simulink model "pde"  (Simulink 6.5)
settings: Solver=ode45  StartTime=0.0  StopTime=10.0  RelTol=1e-3
undefined symbols (not defined in the file): dfilt
libraries: dsparch4 x158, cdsEpicsOut x39, cdsMatrix x11, cdsSwitch x5, cdsWD x5, cdsWfsPhase x4, cdsEpicsIn x4, dac x2, cdsRemoteIntlk x1, cdsParameters x1
(part 2 of 3)

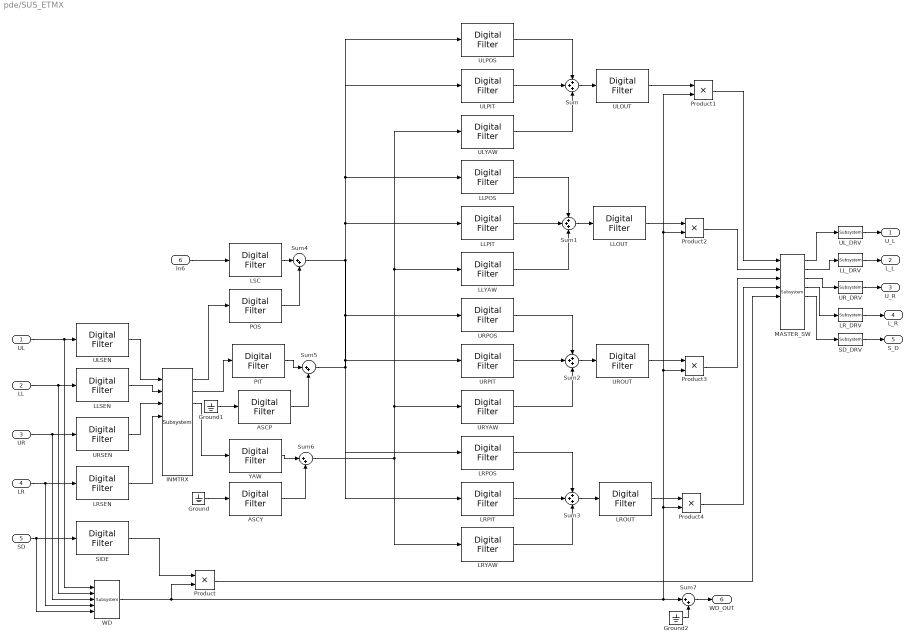
== system pde/SUS_ETMX ==
  UL : Inport
  LL : Inport  Port=2
  UR : Inport  Port=3
  LR : Inport  Port=4
  SD : Inport  Port=5
  In6 : Inport  Port=6
  ASCP : dsparch4/Digital Filter  DialogController=dspdialog.DigitalFilter  DialogControllerArgs=DataTag50  TypePopup=IIR (poles & zeros)  IIRFiltStruct=Direct form II transposed  AllPoleFiltStruct=Direct form  FIRFiltStruct=Direct form  CoeffSource=Specify via dialog  NumCoeffs=[1 2]  DenCoeffs=[1 0.1]  BiQuadCoeffs=[1 0.3 0.4 1 0.1 0.2]  LatticeCoeffs=[0.2 0.4]  denIgnore=on  FiltPerSampPopup=One filter per frame  IC=0  ICnum=0  ICden=0  roundingMode=Floor  overflowMode=off  ScaleValues=1  scaleValueFracLength=14  stageInFracLength=15  stageOutFracLength=15  FilterSource=Specify via dialog  dfiltObjectName=dfilt.dffir([1 2 1])
  ASCY : dsparch4/Digital Filter  DialogController=dspdialog.DigitalFilter  DialogControllerArgs=DataTag51  TypePopup=IIR (poles & zeros)  IIRFiltStruct=Direct form II transposed  AllPoleFiltStruct=Direct form  FIRFiltStruct=Direct form  CoeffSource=Specify via dialog  NumCoeffs=[1 2]  DenCoeffs=[1 0.1]  BiQuadCoeffs=[1 0.3 0.4 1 0.1 0.2]  LatticeCoeffs=[0.2 0.4]  denIgnore=on  FiltPerSampPopup=One filter per frame  IC=0  ICnum=0  ICden=0  roundingMode=Floor  overflowMode=off  ScaleValues=1  scaleValueFracLength=14  stageInFracLength=15  stageOutFracLength=15  FilterSource=Specify via dialog  dfiltObjectName=dfilt.dffir([1 2 1])
  Ground : Ground
  Ground1 : Ground
  Ground2 : Ground
  INMTRX : cdsMatrix/Subsystem  Tag=Matrix  Description=|  SystemSampleTime=-1
      | Purpose:                                                                 
      | Provide a matrix multiplication function for up to 8 input and 8 outputs.
      settings: AttributesFormatString=%<Tag>
  LLOUT : dsparch4/Digital Filter  DialogController=dspdialog.DigitalFilter  DialogControllerArgs=DataTag52  TypePopup=IIR (poles & zeros)  IIRFiltStruct=Direct form II transposed  AllPoleFiltStruct=Direct form  FIRFiltStruct=Direct form  CoeffSource=Specify via dialog  NumCoeffs=[1 2]  DenCoeffs=[1 0.1]  BiQuadCoeffs=[1 0.3 0.4 1 0.1 0.2]  LatticeCoeffs=[0.2 0.4]  denIgnore=on  FiltPerSampPopup=One filter per frame  IC=0  ICnum=0  ICden=0  roundingMode=Floor  overflowMode=off  ScaleValues=1  scaleValueFracLength=14  stageInFracLength=15  stageOutFracLength=15  FilterSource=Specify via dialog  dfiltObjectName=dfilt.dffir([1 2 1])
  LLPIT : dsparch4/Digital Filter  DialogController=dspdialog.DigitalFilter  DialogControllerArgs=DataTag53  TypePopup=IIR (poles & zeros)  IIRFiltStruct=Direct form II transposed  AllPoleFiltStruct=Direct form  FIRFiltStruct=Direct form  CoeffSource=Specify via dialog  NumCoeffs=[1 2]  DenCoeffs=[1 0.1]  BiQuadCoeffs=[1 0.3 0.4 1 0.1 0.2]  LatticeCoeffs=[0.2 0.4]  denIgnore=on  FiltPerSampPopup=One filter per frame  IC=0  ICnum=0  ICden=0  roundingMode=Floor  overflowMode=off  ScaleValues=1  scaleValueFracLength=14  stageInFracLength=15  stageOutFracLength=15  FilterSource=Specify via dialog  dfiltObjectName=dfilt.dffir([1 2 1])
  LLPOS : dsparch4/Digital Filter  DialogController=dspdialog.DigitalFilter  DialogControllerArgs=DataTag54  TypePopup=IIR (poles & zeros)  IIRFiltStruct=Direct form II transposed  AllPoleFiltStruct=Direct form  FIRFiltStruct=Direct form  CoeffSource=Specify via dialog  NumCoeffs=[1 2]  DenCoeffs=[1 0.1]  BiQuadCoeffs=[1 0.3 0.4 1 0.1 0.2]  LatticeCoeffs=[0.2 0.4]  denIgnore=on  FiltPerSampPopup=One filter per frame  IC=0  ICnum=0  ICden=0  roundingMode=Floor  overflowMode=off  ScaleValues=1  scaleValueFracLength=14  stageInFracLength=15  stageOutFracLength=15  FilterSource=Specify via dialog  dfiltObjectName=dfilt.dffir([1 2 1])
  LLSEN : dsparch4/Digital Filter  DialogController=dspdialog.DigitalFilter  DialogControllerArgs=DataTag55  TypePopup=IIR (poles & zeros)  IIRFiltStruct=Direct form II transposed  AllPoleFiltStruct=Direct form  FIRFiltStruct=Direct form  CoeffSource=Specify via dialog  NumCoeffs=[1 2]  DenCoeffs=[1 0.1]  BiQuadCoeffs=[1 0.3 0.4 1 0.1 0.2]  LatticeCoeffs=[0.2 0.4]  denIgnore=on  FiltPerSampPopup=One filter per frame  IC=0  ICnum=0  ICden=0  roundingMode=Floor  overflowMode=off  ScaleValues=1  scaleValueFracLength=14  stageInFracLength=15  stageOutFracLength=15  FilterSource=Specify via dialog  dfiltObjectName=dfilt.dffir([1 2 1])
  LLYAW : dsparch4/Digital Filter  DialogController=dspdialog.DigitalFilter  DialogControllerArgs=DataTag56  TypePopup=IIR (poles & zeros)  IIRFiltStruct=Direct form II transposed  AllPoleFiltStruct=Direct form  FIRFiltStruct=Direct form  CoeffSource=Specify via dialog  NumCoeffs=[1 2]  DenCoeffs=[1 0.1]  BiQuadCoeffs=[1 0.3 0.4 1 0.1 0.2]  LatticeCoeffs=[0.2 0.4]  denIgnore=on  FiltPerSampPopup=One filter per frame  IC=0  ICnum=0  ICden=0  roundingMode=Floor  overflowMode=off  ScaleValues=1  scaleValueFracLength=14  stageInFracLength=15  stageOutFracLength=15  FilterSource=Specify via dialog  dfiltObjectName=dfilt.dffir([1 2 1])
  LL_DRV : cdsEpicsOut/Subsystem  SystemSampleTime=-1
  LROUT : dsparch4/Digital Filter  DialogController=dspdialog.DigitalFilter  DialogControllerArgs=DataTag57  TypePopup=IIR (poles & zeros)  IIRFiltStruct=Direct form II transposed  AllPoleFiltStruct=Direct form  FIRFiltStruct=Direct form  CoeffSource=Specify via dialog  NumCoeffs=[1 2]  DenCoeffs=[1 0.1]  BiQuadCoeffs=[1 0.3 0.4 1 0.1 0.2]  LatticeCoeffs=[0.2 0.4]  denIgnore=on  FiltPerSampPopup=One filter per frame  IC=0  ICnum=0  ICden=0  roundingMode=Floor  overflowMode=off  ScaleValues=1  scaleValueFracLength=14  stageInFracLength=15  stageOutFracLength=15  FilterSource=Specify via dialog  dfiltObjectName=dfilt.dffir([1 2 1])
  LRPIT : dsparch4/Digital Filter  DialogController=dspdialog.DigitalFilter  DialogControllerArgs=DataTag58  TypePopup=IIR (poles & zeros)  IIRFiltStruct=Direct form II transposed  AllPoleFiltStruct=Direct form  FIRFiltStruct=Direct form  CoeffSource=Specify via dialog  NumCoeffs=[1 2]  DenCoeffs=[1 0.1]  BiQuadCoeffs=[1 0.3 0.4 1 0.1 0.2]  LatticeCoeffs=[0.2 0.4]  denIgnore=on  FiltPerSampPopup=One filter per frame  IC=0  ICnum=0  ICden=0  roundingMode=Floor  overflowMode=off  ScaleValues=1  scaleValueFracLength=14  stageInFracLength=15  stageOutFracLength=15  FilterSource=Specify via dialog  dfiltObjectName=dfilt.dffir([1 2 1])
  LRPOS : dsparch4/Digital Filter  DialogController=dspdialog.DigitalFilter  DialogControllerArgs=DataTag59  TypePopup=IIR (poles & zeros)  IIRFiltStruct=Direct form II transposed  AllPoleFiltStruct=Direct form  FIRFiltStruct=Direct form  CoeffSource=Specify via dialog  NumCoeffs=[1 2]  DenCoeffs=[1 0.1]  BiQuadCoeffs=[1 0.3 0.4 1 0.1 0.2]  LatticeCoeffs=[0.2 0.4]  denIgnore=on  FiltPerSampPopup=One filter per frame  IC=0  ICnum=0  ICden=0  roundingMode=Floor  overflowMode=off  ScaleValues=1  scaleValueFracLength=14  stageInFracLength=15  stageOutFracLength=15  FilterSource=Specify via dialog  dfiltObjectName=dfilt.dffir([1 2 1])
  LRSEN : dsparch4/Digital Filter  DialogController=dspdialog.DigitalFilter  DialogControllerArgs=DataTag60  TypePopup=IIR (poles & zeros)  IIRFiltStruct=Direct form II transposed  AllPoleFiltStruct=Direct form  FIRFiltStruct=Direct form  CoeffSource=Specify via dialog  NumCoeffs=[1 2]  DenCoeffs=[1 0.1]  BiQuadCoeffs=[1 0.3 0.4 1 0.1 0.2]  LatticeCoeffs=[0.2 0.4]  denIgnore=on  FiltPerSampPopup=One filter per frame  IC=0  ICnum=0  ICden=0  roundingMode=Floor  overflowMode=off  ScaleValues=1  scaleValueFracLength=14  stageInFracLength=15  stageOutFracLength=15  FilterSource=Specify via dialog  dfiltObjectName=dfilt.dffir([1 2 1])
  LRYAW : dsparch4/Digital Filter  DialogController=dspdialog.DigitalFilter  DialogControllerArgs=DataTag61  TypePopup=IIR (poles & zeros)  IIRFiltStruct=Direct form II transposed  AllPoleFiltStruct=Direct form  FIRFiltStruct=Direct form  CoeffSource=Specify via dialog  NumCoeffs=[1 2]  DenCoeffs=[1 0.1]  BiQuadCoeffs=[1 0.3 0.4 1 0.1 0.2]  LatticeCoeffs=[0.2 0.4]  denIgnore=on  FiltPerSampPopup=One filter per frame  IC=0  ICnum=0  ICden=0  roundingMode=Floor  overflowMode=off  ScaleValues=1  scaleValueFracLength=14  stageInFracLength=15  stageOutFracLength=15  FilterSource=Specify via dialog  dfiltObjectName=dfilt.dffir([1 2 1])
  LR_DRV : cdsEpicsOut/Subsystem  SystemSampleTime=-1
  LSC : dsparch4/Digital Filter  DialogController=dspdialog.DigitalFilter  DialogControllerArgs=DataTag62  TypePopup=IIR (poles & zeros)  IIRFiltStruct=Direct form II transposed  AllPoleFiltStruct=Direct form  FIRFiltStruct=Direct form  CoeffSource=Specify via dialog  NumCoeffs=[1 2]  DenCoeffs=[1 0.1]  BiQuadCoeffs=[1 0.3 0.4 1 0.1 0.2]  LatticeCoeffs=[0.2 0.4]  denIgnore=on  FiltPerSampPopup=One filter per frame  IC=0  ICnum=0  ICden=0  roundingMode=Floor  overflowMode=off  ScaleValues=1  scaleValueFracLength=14  stageInFracLength=15  stageOutFracLength=15  FilterSource=Specify via dialog  dfiltObjectName=dfilt.dffir([1 2 1])
  MASTER_SW : cdsSwitch/Subsystem  SystemSampleTime=-1
  PIT : dsparch4/Digital Filter  DialogController=dspdialog.DigitalFilter  DialogControllerArgs=DataTag63  TypePopup=IIR (poles & zeros)  IIRFiltStruct=Direct form II transposed  AllPoleFiltStruct=Direct form  FIRFiltStruct=Direct form  CoeffSource=Specify via dialog  NumCoeffs=[1 2]  DenCoeffs=[1 0.1]  BiQuadCoeffs=[1 0.3 0.4 1 0.1 0.2]  LatticeCoeffs=[0.2 0.4]  denIgnore=on  FiltPerSampPopup=One filter per frame  IC=0  ICnum=0  ICden=0  roundingMode=Floor  overflowMode=off  ScaleValues=1  scaleValueFracLength=14  stageInFracLength=15  stageOutFracLength=15  FilterSource=Specify via dialog  dfiltObjectName=dfilt.dffir([1 2 1])
  POS : dsparch4/Digital Filter  DialogController=dspdialog.DigitalFilter  DialogControllerArgs=DataTag64  TypePopup=IIR (poles & zeros)  IIRFiltStruct=Direct form II transposed  AllPoleFiltStruct=Direct form  FIRFiltStruct=Direct form  CoeffSource=Specify via dialog  NumCoeffs=[1 2]  DenCoeffs=[1 0.1]  BiQuadCoeffs=[1 0.3 0.4 1 0.1 0.2]  LatticeCoeffs=[0.2 0.4]  denIgnore=on  FiltPerSampPopup=One filter per frame  IC=0  ICnum=0  ICden=0  roundingMode=Floor  overflowMode=off  ScaleValues=1  scaleValueFracLength=14  stageInFracLength=15  stageOutFracLength=15  FilterSource=Specify via dialog  dfiltObjectName=dfilt.dffir([1 2 1])
  Product{,1..4} (5 alike) : Product  RndMeth=Zero
  SD_DRV : cdsEpicsOut/Subsystem  SystemSampleTime=-1
  SIDE : dsparch4/Digital Filter  DialogController=dspdialog.DigitalFilter  DialogControllerArgs=DataTag65  TypePopup=IIR (poles & zeros)  IIRFiltStruct=Direct form II transposed  AllPoleFiltStruct=Direct form  FIRFiltStruct=Direct form  CoeffSource=Specify via dialog  NumCoeffs=[1 2]  DenCoeffs=[1 0.1]  BiQuadCoeffs=[1 0.3 0.4 1 0.1 0.2]  LatticeCoeffs=[0.2 0.4]  denIgnore=on  FiltPerSampPopup=One filter per frame  IC=0  ICnum=0  ICden=0  roundingMode=Floor  overflowMode=off  ScaleValues=1  scaleValueFracLength=14  stageInFracLength=15  stageOutFracLength=15  FilterSource=Specify via dialog  dfiltObjectName=dfilt.dffir([1 2 1])
  Sum{,1..3} (4 alike) : Sum  Inputs=+++
  Sum{4..7} (4 alike) : Sum  Inputs=|++
  ULOUT : dsparch4/Digital Filter  DialogController=dspdialog.DigitalFilter  DialogControllerArgs=DataTag66  TypePopup=IIR (poles & zeros)  IIRFiltStruct=Direct form II transposed  AllPoleFiltStruct=Direct form  FIRFiltStruct=Direct form  CoeffSource=Specify via dialog  NumCoeffs=[1 2]  DenCoeffs=[1 0.1]  BiQuadCoeffs=[1 0.3 0.4 1 0.1 0.2]  LatticeCoeffs=[0.2 0.4]  denIgnore=on  FiltPerSampPopup=One filter per frame  IC=0  ICnum=0  ICden=0  roundingMode=Floor  overflowMode=off  ScaleValues=1  scaleValueFracLength=14  stageInFracLength=15  stageOutFracLength=15  FilterSource=Specify via dialog  dfiltObjectName=dfilt.dffir([1 2 1])
  ULPIT : dsparch4/Digital Filter  DialogController=dspdialog.DigitalFilter  DialogControllerArgs=DataTag67  TypePopup=IIR (poles & zeros)  IIRFiltStruct=Direct form II transposed  AllPoleFiltStruct=Direct form  FIRFiltStruct=Direct form  CoeffSource=Specify via dialog  NumCoeffs=[1 2]  DenCoeffs=[1 0.1]  BiQuadCoeffs=[1 0.3 0.4 1 0.1 0.2]  LatticeCoeffs=[0.2 0.4]  denIgnore=on  FiltPerSampPopup=One filter per frame  IC=0  ICnum=0  ICden=0  roundingMode=Floor  overflowMode=off  ScaleValues=1  scaleValueFracLength=14  stageInFracLength=15  stageOutFracLength=15  FilterSource=Specify via dialog  dfiltObjectName=dfilt.dffir([1 2 1])
  ULPOS : dsparch4/Digital Filter  DialogController=dspdialog.DigitalFilter  DialogControllerArgs=DataTag68  TypePopup=IIR (poles & zeros)  IIRFiltStruct=Direct form II transposed  AllPoleFiltStruct=Direct form  FIRFiltStruct=Direct form  CoeffSource=Specify via dialog  NumCoeffs=[1 2]  DenCoeffs=[1 0.1]  BiQuadCoeffs=[1 0.3 0.4 1 0.1 0.2]  LatticeCoeffs=[0.2 0.4]  denIgnore=on  FiltPerSampPopup=One filter per frame  IC=0  ICnum=0  ICden=0  roundingMode=Floor  overflowMode=off  ScaleValues=1  scaleValueFracLength=14  stageInFracLength=15  stageOutFracLength=15  FilterSource=Specify via dialog  dfiltObjectName=dfilt.dffir([1 2 1])
  ULSEN : dsparch4/Digital Filter  DialogController=dspdialog.DigitalFilter  DialogControllerArgs=DataTag69  TypePopup=IIR (poles & zeros)  IIRFiltStruct=Direct form II transposed  AllPoleFiltStruct=Direct form  FIRFiltStruct=Direct form  CoeffSource=Specify via dialog  NumCoeffs=[1 2]  DenCoeffs=[1 0.1]  BiQuadCoeffs=[1 0.3 0.4 1 0.1 0.2]  LatticeCoeffs=[0.2 0.4]  denIgnore=on  FiltPerSampPopup=One filter per frame  IC=0  ICnum=0  ICden=0  roundingMode=Floor  overflowMode=off  ScaleValues=1  scaleValueFracLength=14  stageInFracLength=15  stageOutFracLength=15  FilterSource=Specify via dialog  dfiltObjectName=dfilt.dffir([1 2 1])
  ULYAW : dsparch4/Digital Filter  DialogController=dspdialog.DigitalFilter  DialogControllerArgs=DataTag70  TypePopup=IIR (poles & zeros)  IIRFiltStruct=Direct form II transposed  AllPoleFiltStruct=Direct form  FIRFiltStruct=Direct form  CoeffSource=Specify via dialog  NumCoeffs=[1 2]  DenCoeffs=[1 0.1]  BiQuadCoeffs=[1 0.3 0.4 1 0.1 0.2]  LatticeCoeffs=[0.2 0.4]  denIgnore=on  FiltPerSampPopup=One filter per frame  IC=0  ICnum=0  ICden=0  roundingMode=Floor  overflowMode=off  ScaleValues=1  scaleValueFracLength=14  stageInFracLength=15  stageOutFracLength=15  FilterSource=Specify via dialog  dfiltObjectName=dfilt.dffir([1 2 1])
  UL_DRV : cdsEpicsOut/Subsystem  SystemSampleTime=-1
  UROUT : dsparch4/Digital Filter  DialogController=dspdialog.DigitalFilter  DialogControllerArgs=DataTag71  TypePopup=IIR (poles & zeros)  IIRFiltStruct=Direct form II transposed  AllPoleFiltStruct=Direct form  FIRFiltStruct=Direct form  CoeffSource=Specify via dialog  NumCoeffs=[1 2]  DenCoeffs=[1 0.1]  BiQuadCoeffs=[1 0.3 0.4 1 0.1 0.2]  LatticeCoeffs=[0.2 0.4]  denIgnore=on  FiltPerSampPopup=One filter per frame  IC=0  ICnum=0  ICden=0  roundingMode=Floor  overflowMode=off  ScaleValues=1  scaleValueFracLength=14  stageInFracLength=15  stageOutFracLength=15  FilterSource=Specify via dialog  dfiltObjectName=dfilt.dffir([1 2 1])
  URPIT : dsparch4/Digital Filter  DialogController=dspdialog.DigitalFilter  DialogControllerArgs=DataTag72  TypePopup=IIR (poles & zeros)  IIRFiltStruct=Direct form II transposed  AllPoleFiltStruct=Direct form  FIRFiltStruct=Direct form  CoeffSource=Specify via dialog  NumCoeffs=[1 2]  DenCoeffs=[1 0.1]  BiQuadCoeffs=[1 0.3 0.4 1 0.1 0.2]  LatticeCoeffs=[0.2 0.4]  denIgnore=on  FiltPerSampPopup=One filter per frame  IC=0  ICnum=0  ICden=0  roundingMode=Floor  overflowMode=off  ScaleValues=1  scaleValueFracLength=14  stageInFracLength=15  stageOutFracLength=15  FilterSource=Specify via dialog  dfiltObjectName=dfilt.dffir([1 2 1])
  URPOS : dsparch4/Digital Filter  DialogController=dspdialog.DigitalFilter  DialogControllerArgs=DataTag73  TypePopup=IIR (poles & zeros)  IIRFiltStruct=Direct form II transposed  AllPoleFiltStruct=Direct form  FIRFiltStruct=Direct form  CoeffSource=Specify via dialog  NumCoeffs=[1 2]  DenCoeffs=[1 0.1]  BiQuadCoeffs=[1 0.3 0.4 1 0.1 0.2]  LatticeCoeffs=[0.2 0.4]  denIgnore=on  FiltPerSampPopup=One filter per frame  IC=0  ICnum=0  ICden=0  roundingMode=Floor  overflowMode=off  ScaleValues=1  scaleValueFracLength=14  stageInFracLength=15  stageOutFracLength=15  FilterSource=Specify via dialog  dfiltObjectName=dfilt.dffir([1 2 1])
  URSEN : dsparch4/Digital Filter  DialogController=dspdialog.DigitalFilter  DialogControllerArgs=DataTag74  TypePopup=IIR (poles & zeros)  IIRFiltStruct=Direct form II transposed  AllPoleFiltStruct=Direct form  FIRFiltStruct=Direct form  CoeffSource=Specify via dialog  NumCoeffs=[1 2]  DenCoeffs=[1 0.1]  BiQuadCoeffs=[1 0.3 0.4 1 0.1 0.2]  LatticeCoeffs=[0.2 0.4]  denIgnore=on  FiltPerSampPopup=One filter per frame  IC=0  ICnum=0  ICden=0  roundingMode=Floor  overflowMode=off  ScaleValues=1  scaleValueFracLength=14  stageInFracLength=15  stageOutFracLength=15  FilterSource=Specify via dialog  dfiltObjectName=dfilt.dffir([1 2 1])
  URYAW : dsparch4/Digital Filter  DialogController=dspdialog.DigitalFilter  DialogControllerArgs=DataTag75  TypePopup=IIR (poles & zeros)  IIRFiltStruct=Direct form II transposed  AllPoleFiltStruct=Direct form  FIRFiltStruct=Direct form  CoeffSource=Specify via dialog  NumCoeffs=[1 2]  DenCoeffs=[1 0.1]  BiQuadCoeffs=[1 0.3 0.4 1 0.1 0.2]  LatticeCoeffs=[0.2 0.4]  denIgnore=on  FiltPerSampPopup=One filter per frame  IC=0  ICnum=0  ICden=0  roundingMode=Floor  overflowMode=off  ScaleValues=1  scaleValueFracLength=14  stageInFracLength=15  stageOutFracLength=15  FilterSource=Specify via dialog  dfiltObjectName=dfilt.dffir([1 2 1])
  UR_DRV : cdsEpicsOut/Subsystem  SystemSampleTime=-1
  WD : cdsWD/Subsystem  SystemSampleTime=-1
  YAW : dsparch4/Digital Filter  DialogController=dspdialog.DigitalFilter  DialogControllerArgs=DataTag76  TypePopup=IIR (poles & zeros)  IIRFiltStruct=Direct form II transposed  AllPoleFiltStruct=Direct form  FIRFiltStruct=Direct form  CoeffSource=Specify via dialog  NumCoeffs=[1 2]  DenCoeffs=[1 0.1]  BiQuadCoeffs=[1 0.3 0.4 1 0.1 0.2]  LatticeCoeffs=[0.2 0.4]  denIgnore=on  FiltPerSampPopup=One filter per frame  IC=0  ICnum=0  ICden=0  roundingMode=Floor  overflowMode=off  ScaleValues=1  scaleValueFracLength=14  stageInFracLength=15  stageOutFracLength=15  FilterSource=Specify via dialog  dfiltObjectName=dfilt.dffir([1 2 1])
  U_L : Outport
  L_L : Outport  Port=2
  U_R : Outport  Port=3
  L_R : Outport  Port=4
  S_D : Outport  Port=5
  WD_OUT : Outport  Port=6
  wires:
  ULSEN/1 -> INMTRX/1
  LLSEN/1 -> INMTRX/2
  URSEN/1 -> INMTRX/3
  LRSEN/1 -> INMTRX/4
  INMTRX/1 -> POS/1
  INMTRX/2 -> PIT/1
  INMTRX/3 -> YAW/1
  ULPOS/1 -> Sum/1
  ULPIT/1 -> Sum/2
  ULYAW/1 -> Sum/3
  LLPOS/1 -> Sum1/1
  LLPIT/1 -> Sum1/2
  LLYAW/1 -> Sum1/3
  URPOS/1 -> Sum2/1
  URPIT/1 -> Sum2/2
  URYAW/1 -> Sum2/3
  LRPOS/1 -> Sum3/1
  LRPIT/1 -> Sum3/2
  LRYAW/1 -> Sum3/3
  Sum/1 -> ULOUT/1
  Sum1/1 -> LLOUT/1
  Sum2/1 -> UROUT/1
  Sum3/1 -> LROUT/1
  UL/1 -> ULSEN/1, WD/1
  LL/1 -> LLSEN/1, WD/2
  UR/1 -> URSEN/1, WD/3
  LR/1 -> LRSEN/1, WD/4
  Ground1/1 -> ASCP/1
  In6/1 -> LSC/1
  Ground/1 -> ASCY/1
  LSC/1 -> Sum4/1
  POS/1 -> Sum4/2
  PIT/1 -> Sum5/1
  ASCP/1 -> Sum5/2
  YAW/1 -> Sum6/1
  ASCY/1 -> Sum6/2
  Sum4/1 -> ULPOS/1, LLPOS/1, URPOS/1, LRPOS/1
  Sum5/1 -> ULPIT/1, LLPIT/1, URPIT/1, LRPIT/1
  Sum6/1 -> ULYAW/1, LLYAW/1, URYAW/1, LRYAW/1
  SD/1 -> SIDE/1, WD/5
  WD/1 -> Product/2, Product4/2, Product3/2, Product2/2, Product1/2, Sum7/1
  SIDE/1 -> Product/1
  ULOUT/1 -> Product1/1
  LLOUT/1 -> Product2/1
  UROUT/1 -> Product3/1
  LROUT/1 -> Product4/1
  LL_DRV/1 -> L_L/1
  UL_DRV/1 -> U_L/1
  UR_DRV/1 -> U_R/1
  LR_DRV/1 -> L_R/1
  SD_DRV/1 -> S_D/1
  Product1/1 -> MASTER_SW/1
  Product2/1 -> MASTER_SW/2
  Product3/1 -> MASTER_SW/3
  Product4/1 -> MASTER_SW/4
  Product/1 -> MASTER_SW/5
  MASTER_SW/1 -> UL_DRV/1
  MASTER_SW/2 -> LL_DRV/1
  MASTER_SW/3 -> UR_DRV/1
  MASTER_SW/4 -> LR_DRV/1
  MASTER_SW/5 -> SD_DRV/1
  Sum7/1 -> WD_OUT/1
  Ground2/1 -> Sum7/2

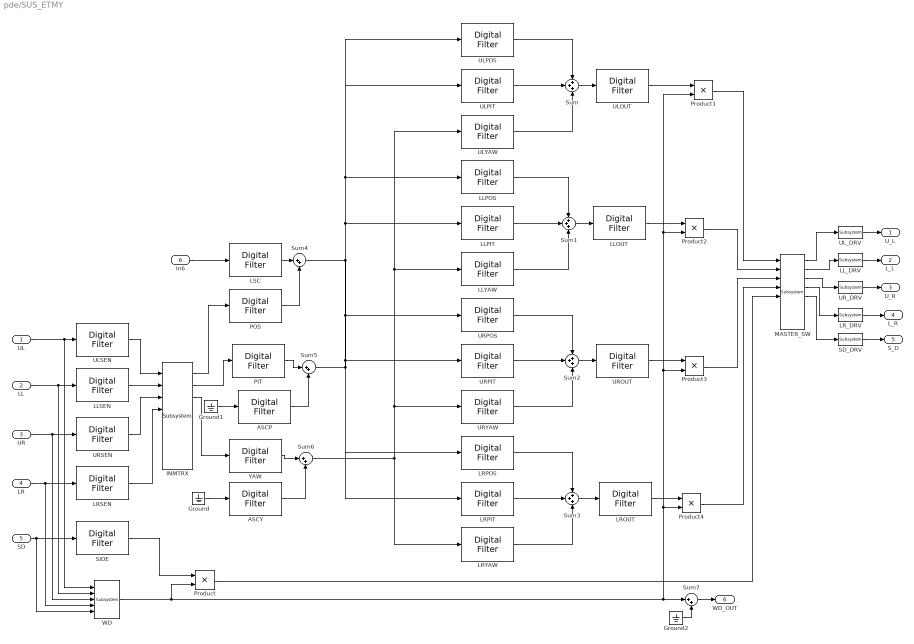
== system pde/SUS_ETMY ==
  UL : Inport
  LL : Inport  Port=2
  UR : Inport  Port=3
  LR : Inport  Port=4
  SD : Inport  Port=5
  In6 : Inport  Port=6
  ASCP : dsparch4/Digital Filter  DialogController=dspdialog.DigitalFilter  DialogControllerArgs=DataTag77  TypePopup=IIR (poles & zeros)  IIRFiltStruct=Direct form II transposed  AllPoleFiltStruct=Direct form  FIRFiltStruct=Direct form  CoeffSource=Specify via dialog  NumCoeffs=[1 2]  DenCoeffs=[1 0.1]  BiQuadCoeffs=[1 0.3 0.4 1 0.1 0.2]  LatticeCoeffs=[0.2 0.4]  denIgnore=on  FiltPerSampPopup=One filter per frame  IC=0  ICnum=0  ICden=0  roundingMode=Floor  overflowMode=off  ScaleValues=1  scaleValueFracLength=14  stageInFracLength=15  stageOutFracLength=15  FilterSource=Specify via dialog  dfiltObjectName=dfilt.dffir([1 2 1])
  ASCY : dsparch4/Digital Filter  DialogController=dspdialog.DigitalFilter  DialogControllerArgs=DataTag78  TypePopup=IIR (poles & zeros)  IIRFiltStruct=Direct form II transposed  AllPoleFiltStruct=Direct form  FIRFiltStruct=Direct form  CoeffSource=Specify via dialog  NumCoeffs=[1 2]  DenCoeffs=[1 0.1]  BiQuadCoeffs=[1 0.3 0.4 1 0.1 0.2]  LatticeCoeffs=[0.2 0.4]  denIgnore=on  FiltPerSampPopup=One filter per frame  IC=0  ICnum=0  ICden=0  roundingMode=Floor  overflowMode=off  ScaleValues=1  scaleValueFracLength=14  stageInFracLength=15  stageOutFracLength=15  FilterSource=Specify via dialog  dfiltObjectName=dfilt.dffir([1 2 1])
  Ground : Ground
  Ground1 : Ground
  Ground2 : Ground
  INMTRX : cdsMatrix/Subsystem  Tag=Matrix  Description=|  SystemSampleTime=-1
      | Purpose:                                                                 
      | Provide a matrix multiplication function for up to 8 input and 8 outputs.
      settings: AttributesFormatString=%<Tag>
  LLOUT : dsparch4/Digital Filter  DialogController=dspdialog.DigitalFilter  DialogControllerArgs=DataTag79  TypePopup=IIR (poles & zeros)  IIRFiltStruct=Direct form II transposed  AllPoleFiltStruct=Direct form  FIRFiltStruct=Direct form  CoeffSource=Specify via dialog  NumCoeffs=[1 2]  DenCoeffs=[1 0.1]  BiQuadCoeffs=[1 0.3 0.4 1 0.1 0.2]  LatticeCoeffs=[0.2 0.4]  denIgnore=on  FiltPerSampPopup=One filter per frame  IC=0  ICnum=0  ICden=0  roundingMode=Floor  overflowMode=off  ScaleValues=1  scaleValueFracLength=14  stageInFracLength=15  stageOutFracLength=15  FilterSource=Specify via dialog  dfiltObjectName=dfilt.dffir([1 2 1])
  LLPIT : dsparch4/Digital Filter  DialogController=dspdialog.DigitalFilter  DialogControllerArgs=DataTag80  TypePopup=IIR (poles & zeros)  IIRFiltStruct=Direct form II transposed  AllPoleFiltStruct=Direct form  FIRFiltStruct=Direct form  CoeffSource=Specify via dialog  NumCoeffs=[1 2]  DenCoeffs=[1 0.1]  BiQuadCoeffs=[1 0.3 0.4 1 0.1 0.2]  LatticeCoeffs=[0.2 0.4]  denIgnore=on  FiltPerSampPopup=One filter per frame  IC=0  ICnum=0  ICden=0  roundingMode=Floor  overflowMode=off  ScaleValues=1  scaleValueFracLength=14  stageInFracLength=15  stageOutFracLength=15  FilterSource=Specify via dialog  dfiltObjectName=dfilt.dffir([1 2 1])
  LLPOS : dsparch4/Digital Filter  DialogController=dspdialog.DigitalFilter  DialogControllerArgs=DataTag81  TypePopup=IIR (poles & zeros)  IIRFiltStruct=Direct form II transposed  AllPoleFiltStruct=Direct form  FIRFiltStruct=Direct form  CoeffSource=Specify via dialog  NumCoeffs=[1 2]  DenCoeffs=[1 0.1]  BiQuadCoeffs=[1 0.3 0.4 1 0.1 0.2]  LatticeCoeffs=[0.2 0.4]  denIgnore=on  FiltPerSampPopup=One filter per frame  IC=0  ICnum=0  ICden=0  roundingMode=Floor  overflowMode=off  ScaleValues=1  scaleValueFracLength=14  stageInFracLength=15  stageOutFracLength=15  FilterSource=Specify via dialog  dfiltObjectName=dfilt.dffir([1 2 1])
  LLSEN : dsparch4/Digital Filter  DialogController=dspdialog.DigitalFilter  DialogControllerArgs=DataTag82  TypePopup=IIR (poles & zeros)  IIRFiltStruct=Direct form II transposed  AllPoleFiltStruct=Direct form  FIRFiltStruct=Direct form  CoeffSource=Specify via dialog  NumCoeffs=[1 2]  DenCoeffs=[1 0.1]  BiQuadCoeffs=[1 0.3 0.4 1 0.1 0.2]  LatticeCoeffs=[0.2 0.4]  denIgnore=on  FiltPerSampPopup=One filter per frame  IC=0  ICnum=0  ICden=0  roundingMode=Floor  overflowMode=off  ScaleValues=1  scaleValueFracLength=14  stageInFracLength=15  stageOutFracLength=15  FilterSource=Specify via dialog  dfiltObjectName=dfilt.dffir([1 2 1])
  LLYAW : dsparch4/Digital Filter  DialogController=dspdialog.DigitalFilter  DialogControllerArgs=DataTag83  TypePopup=IIR (poles & zeros)  IIRFiltStruct=Direct form II transposed  AllPoleFiltStruct=Direct form  FIRFiltStruct=Direct form  CoeffSource=Specify via dialog  NumCoeffs=[1 2]  DenCoeffs=[1 0.1]  BiQuadCoeffs=[1 0.3 0.4 1 0.1 0.2]  LatticeCoeffs=[0.2 0.4]  denIgnore=on  FiltPerSampPopup=One filter per frame  IC=0  ICnum=0  ICden=0  roundingMode=Floor  overflowMode=off  ScaleValues=1  scaleValueFracLength=14  stageInFracLength=15  stageOutFracLength=15  FilterSource=Specify via dialog  dfiltObjectName=dfilt.dffir([1 2 1])
  LL_DRV : cdsEpicsOut/Subsystem  SystemSampleTime=-1
  LROUT : dsparch4/Digital Filter  DialogController=dspdialog.DigitalFilter  DialogControllerArgs=DataTag84  TypePopup=IIR (poles & zeros)  IIRFiltStruct=Direct form II transposed  AllPoleFiltStruct=Direct form  FIRFiltStruct=Direct form  CoeffSource=Specify via dialog  NumCoeffs=[1 2]  DenCoeffs=[1 0.1]  BiQuadCoeffs=[1 0.3 0.4 1 0.1 0.2]  LatticeCoeffs=[0.2 0.4]  denIgnore=on  FiltPerSampPopup=One filter per frame  IC=0  ICnum=0  ICden=0  roundingMode=Floor  overflowMode=off  ScaleValues=1  scaleValueFracLength=14  stageInFracLength=15  stageOutFracLength=15  FilterSource=Specify via dialog  dfiltObjectName=dfilt.dffir([1 2 1])
  LRPIT : dsparch4/Digital Filter  DialogController=dspdialog.DigitalFilter  DialogControllerArgs=DataTag85  TypePopup=IIR (poles & zeros)  IIRFiltStruct=Direct form II transposed  AllPoleFiltStruct=Direct form  FIRFiltStruct=Direct form  CoeffSource=Specify via dialog  NumCoeffs=[1 2]  DenCoeffs=[1 0.1]  BiQuadCoeffs=[1 0.3 0.4 1 0.1 0.2]  LatticeCoeffs=[0.2 0.4]  denIgnore=on  FiltPerSampPopup=One filter per frame  IC=0  ICnum=0  ICden=0  roundingMode=Floor  overflowMode=off  ScaleValues=1  scaleValueFracLength=14  stageInFracLength=15  stageOutFracLength=15  FilterSource=Specify via dialog  dfiltObjectName=dfilt.dffir([1 2 1])
  LRPOS : dsparch4/Digital Filter  DialogController=dspdialog.DigitalFilter  DialogControllerArgs=DataTag86  TypePopup=IIR (poles & zeros)  IIRFiltStruct=Direct form II transposed  AllPoleFiltStruct=Direct form  FIRFiltStruct=Direct form  CoeffSource=Specify via dialog  NumCoeffs=[1 2]  DenCoeffs=[1 0.1]  BiQuadCoeffs=[1 0.3 0.4 1 0.1 0.2]  LatticeCoeffs=[0.2 0.4]  denIgnore=on  FiltPerSampPopup=One filter per frame  IC=0  ICnum=0  ICden=0  roundingMode=Floor  overflowMode=off  ScaleValues=1  scaleValueFracLength=14  stageInFracLength=15  stageOutFracLength=15  FilterSource=Specify via dialog  dfiltObjectName=dfilt.dffir([1 2 1])
  LRSEN : dsparch4/Digital Filter  DialogController=dspdialog.DigitalFilter  DialogControllerArgs=DataTag87  TypePopup=IIR (poles & zeros)  IIRFiltStruct=Direct form II transposed  AllPoleFiltStruct=Direct form  FIRFiltStruct=Direct form  CoeffSource=Specify via dialog  NumCoeffs=[1 2]  DenCoeffs=[1 0.1]  BiQuadCoeffs=[1 0.3 0.4 1 0.1 0.2]  LatticeCoeffs=[0.2 0.4]  denIgnore=on  FiltPerSampPopup=One filter per frame  IC=0  ICnum=0  ICden=0  roundingMode=Floor  overflowMode=off  ScaleValues=1  scaleValueFracLength=14  stageInFracLength=15  stageOutFracLength=15  FilterSource=Specify via dialog  dfiltObjectName=dfilt.dffir([1 2 1])
  LRYAW : dsparch4/Digital Filter  DialogController=dspdialog.DigitalFilter  DialogControllerArgs=DataTag88  TypePopup=IIR (poles & zeros)  IIRFiltStruct=Direct form II transposed  AllPoleFiltStruct=Direct form  FIRFiltStruct=Direct form  CoeffSource=Specify via dialog  NumCoeffs=[1 2]  DenCoeffs=[1 0.1]  BiQuadCoeffs=[1 0.3 0.4 1 0.1 0.2]  LatticeCoeffs=[0.2 0.4]  denIgnore=on  FiltPerSampPopup=One filter per frame  IC=0  ICnum=0  ICden=0  roundingMode=Floor  overflowMode=off  ScaleValues=1  scaleValueFracLength=14  stageInFracLength=15  stageOutFracLength=15  FilterSource=Specify via dialog  dfiltObjectName=dfilt.dffir([1 2 1])
  LR_DRV : cdsEpicsOut/Subsystem  SystemSampleTime=-1
  LSC : dsparch4/Digital Filter  DialogController=dspdialog.DigitalFilter  DialogControllerArgs=DataTag89  TypePopup=IIR (poles & zeros)  IIRFiltStruct=Direct form II transposed  AllPoleFiltStruct=Direct form  FIRFiltStruct=Direct form  CoeffSource=Specify via dialog  NumCoeffs=[1 2]  DenCoeffs=[1 0.1]  BiQuadCoeffs=[1 0.3 0.4 1 0.1 0.2]  LatticeCoeffs=[0.2 0.4]  denIgnore=on  FiltPerSampPopup=One filter per frame  IC=0  ICnum=0  ICden=0  roundingMode=Floor  overflowMode=off  ScaleValues=1  scaleValueFracLength=14  stageInFracLength=15  stageOutFracLength=15  FilterSource=Specify via dialog  dfiltObjectName=dfilt.dffir([1 2 1])
  MASTER_SW : cdsSwitch/Subsystem  SystemSampleTime=-1
  PIT : dsparch4/Digital Filter  DialogController=dspdialog.DigitalFilter  DialogControllerArgs=DataTag90  TypePopup=IIR (poles & zeros)  IIRFiltStruct=Direct form II transposed  AllPoleFiltStruct=Direct form  FIRFiltStruct=Direct form  CoeffSource=Specify via dialog  NumCoeffs=[1 2]  DenCoeffs=[1 0.1]  BiQuadCoeffs=[1 0.3 0.4 1 0.1 0.2]  LatticeCoeffs=[0.2 0.4]  denIgnore=on  FiltPerSampPopup=One filter per frame  IC=0  ICnum=0  ICden=0  roundingMode=Floor  overflowMode=off  ScaleValues=1  scaleValueFracLength=14  stageInFracLength=15  stageOutFracLength=15  FilterSource=Specify via dialog  dfiltObjectName=dfilt.dffir([1 2 1])
  POS : dsparch4/Digital Filter  DialogController=dspdialog.DigitalFilter  DialogControllerArgs=DataTag91  TypePopup=IIR (poles & zeros)  IIRFiltStruct=Direct form II transposed  AllPoleFiltStruct=Direct form  FIRFiltStruct=Direct form  CoeffSource=Specify via dialog  NumCoeffs=[1 2]  DenCoeffs=[1 0.1]  BiQuadCoeffs=[1 0.3 0.4 1 0.1 0.2]  LatticeCoeffs=[0.2 0.4]  denIgnore=on  FiltPerSampPopup=One filter per frame  IC=0  ICnum=0  ICden=0  roundingMode=Floor  overflowMode=off  ScaleValues=1  scaleValueFracLength=14  stageInFracLength=15  stageOutFracLength=15  FilterSource=Specify via dialog  dfiltObjectName=dfilt.dffir([1 2 1])
  Product{,1..4} (5 alike) : Product  RndMeth=Zero
  SD_DRV : cdsEpicsOut/Subsystem  SystemSampleTime=-1
  SIDE : dsparch4/Digital Filter  DialogController=dspdialog.DigitalFilter  DialogControllerArgs=DataTag92  TypePopup=IIR (poles & zeros)  IIRFiltStruct=Direct form II transposed  AllPoleFiltStruct=Direct form  FIRFiltStruct=Direct form  CoeffSource=Specify via dialog  NumCoeffs=[1 2]  DenCoeffs=[1 0.1]  BiQuadCoeffs=[1 0.3 0.4 1 0.1 0.2]  LatticeCoeffs=[0.2 0.4]  denIgnore=on  FiltPerSampPopup=One filter per frame  IC=0  ICnum=0  ICden=0  roundingMode=Floor  overflowMode=off  ScaleValues=1  scaleValueFracLength=14  stageInFracLength=15  stageOutFracLength=15  FilterSource=Specify via dialog  dfiltObjectName=dfilt.dffir([1 2 1])
  Sum{,1..3} (4 alike) : Sum  Inputs=+++
  Sum{4..7} (4 alike) : Sum  Inputs=|++
  ULOUT : dsparch4/Digital Filter  DialogController=dspdialog.DigitalFilter  DialogControllerArgs=DataTag93  TypePopup=IIR (poles & zeros)  IIRFiltStruct=Direct form II transposed  AllPoleFiltStruct=Direct form  FIRFiltStruct=Direct form  CoeffSource=Specify via dialog  NumCoeffs=[1 2]  DenCoeffs=[1 0.1]  BiQuadCoeffs=[1 0.3 0.4 1 0.1 0.2]  LatticeCoeffs=[0.2 0.4]  denIgnore=on  FiltPerSampPopup=One filter per frame  IC=0  ICnum=0  ICden=0  roundingMode=Floor  overflowMode=off  ScaleValues=1  scaleValueFracLength=14  stageInFracLength=15  stageOutFracLength=15  FilterSource=Specify via dialog  dfiltObjectName=dfilt.dffir([1 2 1])
  ULPIT : dsparch4/Digital Filter  DialogController=dspdialog.DigitalFilter  DialogControllerArgs=DataTag94  TypePopup=IIR (poles & zeros)  IIRFiltStruct=Direct form II transposed  AllPoleFiltStruct=Direct form  FIRFiltStruct=Direct form  CoeffSource=Specify via dialog  NumCoeffs=[1 2]  DenCoeffs=[1 0.1]  BiQuadCoeffs=[1 0.3 0.4 1 0.1 0.2]  LatticeCoeffs=[0.2 0.4]  denIgnore=on  FiltPerSampPopup=One filter per frame  IC=0  ICnum=0  ICden=0  roundingMode=Floor  overflowMode=off  ScaleValues=1  scaleValueFracLength=14  stageInFracLength=15  stageOutFracLength=15  FilterSource=Specify via dialog  dfiltObjectName=dfilt.dffir([1 2 1])
  ULPOS : dsparch4/Digital Filter  DialogController=dspdialog.DigitalFilter  DialogControllerArgs=DataTag95  TypePopup=IIR (poles & zeros)  IIRFiltStruct=Direct form II transposed  AllPoleFiltStruct=Direct form  FIRFiltStruct=Direct form  CoeffSource=Specify via dialog  NumCoeffs=[1 2]  DenCoeffs=[1 0.1]  BiQuadCoeffs=[1 0.3 0.4 1 0.1 0.2]  LatticeCoeffs=[0.2 0.4]  denIgnore=on  FiltPerSampPopup=One filter per frame  IC=0  ICnum=0  ICden=0  roundingMode=Floor  overflowMode=off  ScaleValues=1  scaleValueFracLength=14  stageInFracLength=15  stageOutFracLength=15  FilterSource=Specify via dialog  dfiltObjectName=dfilt.dffir([1 2 1])
  ULSEN : dsparch4/Digital Filter  DialogController=dspdialog.DigitalFilter  DialogControllerArgs=DataTag96  TypePopup=IIR (poles & zeros)  IIRFiltStruct=Direct form II transposed  AllPoleFiltStruct=Direct form  FIRFiltStruct=Direct form  CoeffSource=Specify via dialog  NumCoeffs=[1 2]  DenCoeffs=[1 0.1]  BiQuadCoeffs=[1 0.3 0.4 1 0.1 0.2]  LatticeCoeffs=[0.2 0.4]  denIgnore=on  FiltPerSampPopup=One filter per frame  IC=0  ICnum=0  ICden=0  roundingMode=Floor  overflowMode=off  ScaleValues=1  scaleValueFracLength=14  stageInFracLength=15  stageOutFracLength=15  FilterSource=Specify via dialog  dfiltObjectName=dfilt.dffir([1 2 1])
  ULYAW : dsparch4/Digital Filter  DialogController=dspdialog.DigitalFilter  DialogControllerArgs=DataTag97  TypePopup=IIR (poles & zeros)  IIRFiltStruct=Direct form II transposed  AllPoleFiltStruct=Direct form  FIRFiltStruct=Direct form  CoeffSource=Specify via dialog  NumCoeffs=[1 2]  DenCoeffs=[1 0.1]  BiQuadCoeffs=[1 0.3 0.4 1 0.1 0.2]  LatticeCoeffs=[0.2 0.4]  denIgnore=on  FiltPerSampPopup=One filter per frame  IC=0  ICnum=0  ICden=0  roundingMode=Floor  overflowMode=off  ScaleValues=1  scaleValueFracLength=14  stageInFracLength=15  stageOutFracLength=15  FilterSource=Specify via dialog  dfiltObjectName=dfilt.dffir([1 2 1])
  UL_DRV : cdsEpicsOut/Subsystem  SystemSampleTime=-1
  UROUT : dsparch4/Digital Filter  DialogController=dspdialog.DigitalFilter  DialogControllerArgs=DataTag98  TypePopup=IIR (poles & zeros)  IIRFiltStruct=Direct form II transposed  AllPoleFiltStruct=Direct form  FIRFiltStruct=Direct form  CoeffSource=Specify via dialog  NumCoeffs=[1 2]  DenCoeffs=[1 0.1]  BiQuadCoeffs=[1 0.3 0.4 1 0.1 0.2]  LatticeCoeffs=[0.2 0.4]  denIgnore=on  FiltPerSampPopup=One filter per frame  IC=0  ICnum=0  ICden=0  roundingMode=Floor  overflowMode=off  ScaleValues=1  scaleValueFracLength=14  stageInFracLength=15  stageOutFracLength=15  FilterSource=Specify via dialog  dfiltObjectName=dfilt.dffir([1 2 1])
  URPIT : dsparch4/Digital Filter  DialogController=dspdialog.DigitalFilter  DialogControllerArgs=DataTag99  TypePopup=IIR (poles & zeros)  IIRFiltStruct=Direct form II transposed  AllPoleFiltStruct=Direct form  FIRFiltStruct=Direct form  CoeffSource=Specify via dialog  NumCoeffs=[1 2]  DenCoeffs=[1 0.1]  BiQuadCoeffs=[1 0.3 0.4 1 0.1 0.2]  LatticeCoeffs=[0.2 0.4]  denIgnore=on  FiltPerSampPopup=One filter per frame  IC=0  ICnum=0  ICden=0  roundingMode=Floor  overflowMode=off  ScaleValues=1  scaleValueFracLength=14  stageInFracLength=15  stageOutFracLength=15  FilterSource=Specify via dialog  dfiltObjectName=dfilt.dffir([1 2 1])
  URPOS : dsparch4/Digital Filter  DialogController=dspdialog.DigitalFilter  DialogControllerArgs=DataTag100  TypePopup=IIR (poles & zeros)  IIRFiltStruct=Direct form II transposed  AllPoleFiltStruct=Direct form  FIRFiltStruct=Direct form  CoeffSource=Specify via dialog  NumCoeffs=[1 2]  DenCoeffs=[1 0.1]  BiQuadCoeffs=[1 0.3 0.4 1 0.1 0.2]  LatticeCoeffs=[0.2 0.4]  denIgnore=on  FiltPerSampPopup=One filter per frame  IC=0  ICnum=0  ICden=0  roundingMode=Floor  overflowMode=off  ScaleValues=1  scaleValueFracLength=14  stageInFracLength=15  stageOutFracLength=15  FilterSource=Specify via dialog  dfiltObjectName=dfilt.dffir([1 2 1])
  URSEN : dsparch4/Digital Filter  DialogController=dspdialog.DigitalFilter  DialogControllerArgs=DataTag101  TypePopup=IIR (poles & zeros)  IIRFiltStruct=Direct form II transposed  AllPoleFiltStruct=Direct form  FIRFiltStruct=Direct form  CoeffSource=Specify via dialog  NumCoeffs=[1 2]  DenCoeffs=[1 0.1]  BiQuadCoeffs=[1 0.3 0.4 1 0.1 0.2]  LatticeCoeffs=[0.2 0.4]  denIgnore=on  FiltPerSampPopup=One filter per frame  IC=0  ICnum=0  ICden=0  roundingMode=Floor  overflowMode=off  ScaleValues=1  scaleValueFracLength=14  stageInFracLength=15  stageOutFracLength=15  FilterSource=Specify via dialog  dfiltObjectName=dfilt.dffir([1 2 1])
  URYAW : dsparch4/Digital Filter  DialogController=dspdialog.DigitalFilter  DialogControllerArgs=DataTag102  TypePopup=IIR (poles & zeros)  IIRFiltStruct=Direct form II transposed  AllPoleFiltStruct=Direct form  FIRFiltStruct=Direct form  CoeffSource=Specify via dialog  NumCoeffs=[1 2]  DenCoeffs=[1 0.1]  BiQuadCoeffs=[1 0.3 0.4 1 0.1 0.2]  LatticeCoeffs=[0.2 0.4]  denIgnore=on  FiltPerSampPopup=One filter per frame  IC=0  ICnum=0  ICden=0  roundingMode=Floor  overflowMode=off  ScaleValues=1  scaleValueFracLength=14  stageInFracLength=15  stageOutFracLength=15  FilterSource=Specify via dialog  dfiltObjectName=dfilt.dffir([1 2 1])
  UR_DRV : cdsEpicsOut/Subsystem  SystemSampleTime=-1
  WD : cdsWD/Subsystem  SystemSampleTime=-1
  YAW : dsparch4/Digital Filter  DialogController=dspdialog.DigitalFilter  DialogControllerArgs=DataTag103  TypePopup=IIR (poles & zeros)  IIRFiltStruct=Direct form II transposed  AllPoleFiltStruct=Direct form  FIRFiltStruct=Direct form  CoeffSource=Specify via dialog  NumCoeffs=[1 2]  DenCoeffs=[1 0.1]  BiQuadCoeffs=[1 0.3 0.4 1 0.1 0.2]  LatticeCoeffs=[0.2 0.4]  denIgnore=on  FiltPerSampPopup=One filter per frame  IC=0  ICnum=0  ICden=0  roundingMode=Floor  overflowMode=off  ScaleValues=1  scaleValueFracLength=14  stageInFracLength=15  stageOutFracLength=15  FilterSource=Specify via dialog  dfiltObjectName=dfilt.dffir([1 2 1])
  U_L : Outport
  L_L : Outport  Port=2
  U_R : Outport  Port=3
  L_R : Outport  Port=4
  S_D : Outport  Port=5
  WD_OUT : Outport  Port=6
  wires:
  ULSEN/1 -> INMTRX/1
  LLSEN/1 -> INMTRX/2
  URSEN/1 -> INMTRX/3
  LRSEN/1 -> INMTRX/4
  INMTRX/1 -> POS/1
  INMTRX/2 -> PIT/1
  INMTRX/3 -> YAW/1
  ULPOS/1 -> Sum/1
  ULPIT/1 -> Sum/2
  ULYAW/1 -> Sum/3
  LLPOS/1 -> Sum1/1
  LLPIT/1 -> Sum1/2
  LLYAW/1 -> Sum1/3
  URPOS/1 -> Sum2/1
  URPIT/1 -> Sum2/2
  URYAW/1 -> Sum2/3
  LRPOS/1 -> Sum3/1
  LRPIT/1 -> Sum3/2
  LRYAW/1 -> Sum3/3
  Sum/1 -> ULOUT/1
  Sum1/1 -> LLOUT/1
  Sum2/1 -> UROUT/1
  Sum3/1 -> LROUT/1
  UL/1 -> ULSEN/1, WD/1
  LL/1 -> LLSEN/1, WD/2
  UR/1 -> URSEN/1, WD/3
  LR/1 -> LRSEN/1, WD/4
  Ground1/1 -> ASCP/1
  In6/1 -> LSC/1
  Ground/1 -> ASCY/1
  LSC/1 -> Sum4/1
  POS/1 -> Sum4/2
  PIT/1 -> Sum5/1
  ASCP/1 -> Sum5/2
  YAW/1 -> Sum6/1
  ASCY/1 -> Sum6/2
  Sum4/1 -> ULPOS/1, LLPOS/1, URPOS/1, LRPOS/1
  Sum5/1 -> ULPIT/1, LLPIT/1, URPIT/1, LRPIT/1
  Sum6/1 -> ULYAW/1, LLYAW/1, URYAW/1, LRYAW/1
  SD/1 -> SIDE/1, WD/5
  WD/1 -> Product/2, Product4/2, Product3/2, Product2/2, Product1/2, Sum7/1
  SIDE/1 -> Product/1
  ULOUT/1 -> Product1/1
  LLOUT/1 -> Product2/1
  UROUT/1 -> Product3/1
  LROUT/1 -> Product4/1
  LL_DRV/1 -> L_L/1
  UL_DRV/1 -> U_L/1
  UR_DRV/1 -> U_R/1
  LR_DRV/1 -> L_R/1
  SD_DRV/1 -> S_D/1
  Product1/1 -> MASTER_SW/1
  Product2/1 -> MASTER_SW/2
  Product3/1 -> MASTER_SW/3
  Product4/1 -> MASTER_SW/4
  Product/1 -> MASTER_SW/5
  MASTER_SW/1 -> UL_DRV/1
  MASTER_SW/2 -> LL_DRV/1
  MASTER_SW/3 -> UR_DRV/1
  MASTER_SW/4 -> LR_DRV/1
  MASTER_SW/5 -> SD_DRV/1
  Ground2/1 -> Sum7/2
  Sum7/1 -> WD_OUT/1
